simulink library "Feeder3_lib"  (Simulink 8.1)
settings: Solver=ode45  StartTime=0.0  StopTime=10.0  RelTol=1e-3
values from neighbouring files (symbols this model uses):
  Ts = 100E-6    (= 0.0001)    [BANSHEE_init.m]
undefined symbols (not defined in the file or in its folder): Left, type, V
libraries: cables_lib x14, breaker_lib x11, Load_lib x6, transformer_lib x5, powerlib x5, rtlab x3, ssn_lib x3, fault_lib x1, PQFV_lib x1, HWController_NGCHP_Genset_3p5MVA_lib x1, Motor_InductionMachine_lib x1
settings Model: Creator=re25624  LastModifiedBy=g73labuser

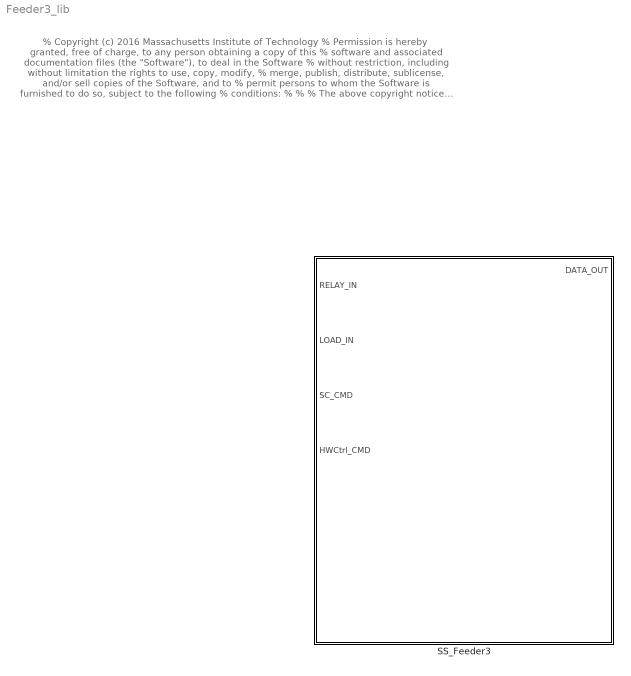
== system Feeder3_lib ==
  note: % Copyright (c) 2016 Massachusetts Institute of Technology
      | % Permission is hereby granted, free of charge, to any person obtaining a copy of this
      | % software and associated documentation files (the "Software"), to deal in the Software
      | % without restriction, including without limitation the rights to use, copy, modify,
      | % merge, publish, distribute, sublicense, and/or sell copies of the Software, and to
      | % permit persons to whom the Software is furnished to do so, subject to the following
      | % conditions:
      | %
      | %
      | % The above copyright notice and this permission notice shall be included in
      | % all copies or substantial portions of the Software.
      | %
      | % THE SOFTWARE IS PROVIDED "AS IS", WITHOUT WARRANTY OF ANY KIND, EXPRESS OR IMPLIED,
      | % INCLUDING BUT NOT LIMITED TO THE WARRANTIES OF MERCHANTABILITY, FITNESS FOR A
      | % PARTICULAR PURPOSE AND NONINFRINGEMENT. IN NO EVENT SHALL THE AUTHORS OR COPYRIGHT
      | % HOLDERS BE LIABLE FOR ANY CLAIM, DAMAGES OR OTHER LIABILITY, WHETHER IN AN ACTION
      | % OF CONTRACT, TORT OR OTHERWISE, ARISING FROM, OUT OF OR IN CONNECTION WITH THE
      | % SOFTWARE OR THE USE OR OTHER DEALINGS IN THE SOFTWARE.
      | %
      | %
      | %%
  SS_Feeder3 : Subsystem

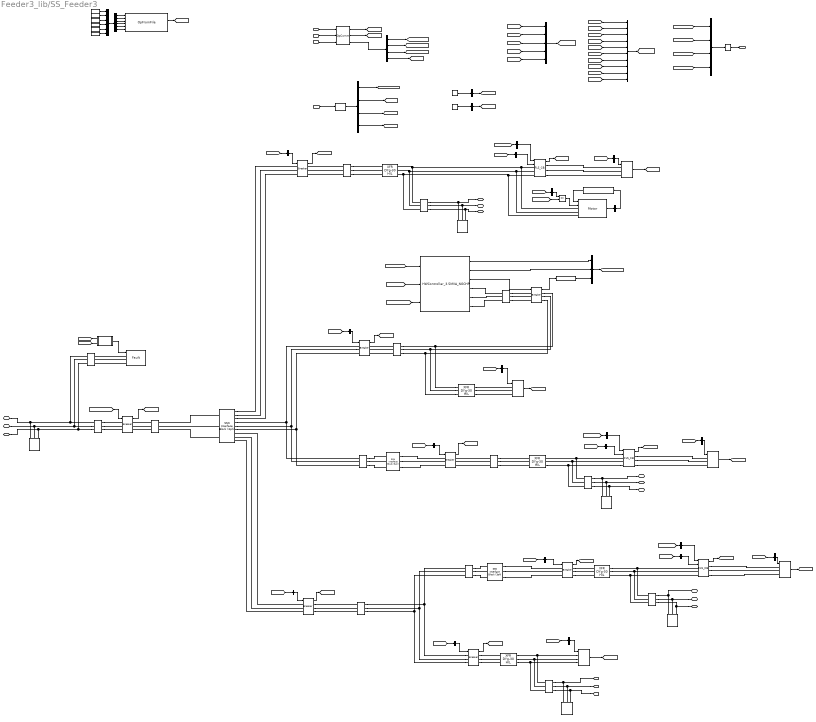
== system Feeder3_lib/SS_Feeder3 ==
  note: % Copyright (c) 2016 Massachusetts Institute of Technology
      | % Permission is hereby granted, free of charge, to any person obtaining a copy of this
      | % software and associated documentation files (the "Software"), to deal in the Software
      | % without restriction, including without limitation the rights to use, copy, modify,
      | % merge, publish, distribute, sublicense, and/or sell copies of the Software, and to
      | % permit persons to whom the Software is furnished to do so, subject to the following
      | % conditions:
      | %
      | %
      | % The above copyright notice and this permission notice shall be included in
      | % all copies or substantial portions of the Software.
      | %
      | % THE SOFTWARE IS PROVIDED "AS IS", WITHOUT WARRANTY OF ANY KIND, EXPRESS OR IMPLIED,
      | % INCLUDING BUT NOT LIMITED TO THE WARRANTIES OF MERCHANTABILITY, FITNESS FOR A
      | % PARTICULAR PURPOSE AND NONINFRINGEMENT. IN NO EVENT SHALL THE AUTHORS OR COPYRIGHT
      | % HOLDERS BE LIABLE FOR ANY CLAIM, DAMAGES OR OTHER LIABILITY, WHETHER IN AN ACTION
      | % OF CONTRACT, TORT OR OTHERWISE, ARISING FROM, OUT OF OR IN CONNECTION WITH THE
      | % SOFTWARE OR THE USE OR OTHER DEALINGS IN THE SOFTWARE.
      | %
      | %
      | %%
  note: connect to F1
  note: connect to F2
  note: connect to F2
  note: connect to F2
  note: Signal for this Cb will come from a SEL relay
  RELAY_IN : Inport
  LOAD_IN : Inport  Port=2
  SC_CMD : Inport  Port=3
  HWCtrl_CMD : Inport  Port=4
  1000 kVA : transformer_lib/XFR DYg-30 HIL  Rating=1000  Vp=13800  Vs=480  Z=5.56  XR=5.49
  1000 kVA1 : transformer_lib/XFR DYg-30 HIL  Rating=1000  Vp=13800  Vs=480  Z=5.56  XR=5.49
  200 HP chiller compressor : Load_lib/200 HP chiller compressor
  2000 kVA : transformer_lib/XFR DYg-30 HIL  Rating=2000  Vp=13800  Vs=480  Z=5.75  XR=5.7
  2000 kVA1 : transformer_lib/XFR DYg-30 HIL  Rating=2000  Vp=13800  Vs=480  Z=5.75  XR=5.7
  2500 kVA : transformer_lib/XFR DYg-30 HIL  Rating=2500  Vp=13800  Vs=480  Z=5.75  XR=6.6
  4/0AWG-Mutual : cables_lib/4//0AWG-Mutual  length=100  par_sets=1  ratio=3
  448 kvar inductor at 13.8kV  to cancel kvar produced by the stublines1 : powerlib/Elements/Three-Phase Parallel RLC Load  LConnTagsString=A|B|C  Configuration=Y (grounded)  NominalVoltage=13800  NominalFrequency=60  ActivePower=0  InductivePower=448e3  CapacitivePower=0  Measurements=None  LoadType=constant Z
  5 kvar inductor at 480V  to cancel kvar produced by the stublines : powerlib/Elements/Three-Phase Parallel RLC Load  LConnTagsString=A|B|C  Configuration=Y (grounded)  NominalVoltage=480  NominalFrequency=60  ActivePower=0  InductivePower=5e3  CapacitivePower=0  Measurements=None  LoadType=constant Z
  500kcmil-Mutual{1..2,4,7,9} (5 alike) : cables_lib/500kcmil-Mutual  length=10  par_sets=1  ratio=3
  500kcmil-Mutual3 : cables_lib/500kcmil-Mutual  length=100  par_sets=1  ratio=3
  500kcmil-Mutual5 : cables_lib/500kcmil-Mutual  length=1000  par_sets=1  ratio=3
  6 kvar inductor at 480V  to cancel kvar produced by the stublines1 : powerlib/Elements/Three-Phase Parallel RLC Load  LConnTagsString=A|B|C  Configuration=Y (grounded)  NominalVoltage=480  NominalFrequency=60  ActivePower=0  InductivePower=6e3  CapacitivePower=0  Measurements=None  LoadType=constant Z
  6 kvar inductor at 480V  to cancel kvar produced by the stublines2 : powerlib/Elements/Three-Phase Parallel RLC Load  LConnTagsString=A|B|C  Configuration=Y (grounded)  NominalVoltage=480  NominalFrequency=60  ActivePower=0  InductivePower=6e3  CapacitivePower=0  Measurements=None  LoadType=constant Z
  6 kvar inductor at 480V  to cancel kvar produced by the stublines3 : powerlib/Elements/Three-Phase Parallel RLC Load  LConnTagsString=A|B|C  Configuration=Y (grounded)  NominalVoltage=480  NominalFrequency=60  ActivePower=0  InductivePower=6e3  CapacitivePower=0  Measurements=None  LoadType=constant Z
  Bus Creator : BusCreator  Inputs=1
  Bus Creator1 : BusCreator  Inputs=1
  Bus Creator2 : BusCreator
  Bus Creator3 : BusCreator  Inputs=5
  Bus Creator5 : BusCreator  Inputs=10
  Bus Creator6 : BusCreator  Inputs=3
  Bus Selector : BusSelector  OutputSignals=motor_2
  Bus Selector1 : BusSelector  OutputSignals=F3_CB_4
  Bus Selector10 : BusSelector  OutputSignals=F3_CB_5
  Bus Selector11 : BusSelector  OutputSignals=P6
  Bus Selector12 : BusSelector  OutputSignals=F3_CB_9
  Bus Selector13 : BusSelector  OutputSignals=F3_CB_3
  Bus Selector14 : BusSelector  OutputSignals=F3_CB_8
  Bus Selector15 : BusSelector  OutputSignals=IO ctrl.16 DOUT GR3.CHP_SIM_Cmds,motor_ONOFF.F3_motor_ONOFF,fault_cmd,GridStatusCtrl.Grid_F3.Logic_trip
  Bus Selector16 : BusSelector  OutputSignals=HWCtrl.NGCHP_Gen1,HWCtrl.SEL751_LogicTrip.F3.Logic_trip,HWCtrl.SEL2440_FLS,TestSeq
  Bus Selector17 : BusSelector  OutputSignals=RPM
  Bus Selector18 : BusSelector  OutputSignals=CB309
  Bus Selector19 : BusSelector  OutputSignals=CB307
  Bus Selector2 : BusSelector  OutputSignals=C6
  Bus Selector20 : BusSelector  OutputSignals=CB308
  Bus Selector3 : BusSelector  OutputSignals=P4
  Bus Selector4 : BusSelector  OutputSignals=I6
  Bus Selector5 : BusSelector  OutputSignals=C5
  Bus Selector6 : BusSelector  OutputSignals=F3_CB_2
  Bus Selector7 : BusSelector  OutputSignals=F3_CB_7
  Bus Selector8 : BusSelector  OutputSignals=F3_CB_6
  Bus Selector9 : BusSelector  OutputSignals=F3_CB_1
  C1 : cables_lib/500kcmil-Mutual  length=10  par_sets=1  ratio=3
  C2 : cables_lib/500kcmil-Mutual  length=10  par_sets=1  ratio=3
  C301 : cables_lib/500kcmil-Mutual  length=2500  par_sets=1  ratio=3
  C302 : cables_lib/4//0AWG-Mutual  length=2000  par_sets=1  ratio=3
  C303 : cables_lib/500kcmil-Mutual  length=2000  par_sets=1  ratio=3
  C304 : cables_lib/4//0AWG-Mutual  length=1500  par_sets=2  ratio=3
  CB closed : Constant
  CB open : Constant  Value=0
  Critical_5 : Load_lib/Dynamic_Load  V=480  kVA=1000  PF=0.9  Ts=Ts
  Critical_6 : Load_lib/Dynamic_Load  V=480  kVA=800  PF=0.9  Ts=Ts
  Demux2 : Demux  Outputs=6
  F3_CB_{1..6} (6 alike) : breaker_lib/Breaker  Ts=Ts  mech_delay=cb_mech_delay
  F3_CB_7 : breaker_lib/FLS_CB  Ts=Ts  mech_delay=cb_mech_delay
  F3_CB_8 : breaker_lib/FLS_CB  Ts=Ts  mech_delay=cb_mech_delay
  F3_CB_9 : breaker_lib/FLS_CB  Ts=Ts  mech_delay=cb_mech_delay
  F3_GCB : breaker_lib/Breaker  Ts=Ts  mech_delay=cb_mech_delay
  F3_PCC : breaker_lib/Breaker  Ts=Ts  mech_delay=cb_mech_delay
  Fault_4 : fault_lib/Fault  FaultResistance=0.5  GroundResistance=1.73  SnubberResistance=1E6
  Genset_PQFV : PQFV_lib/Genset_PQFV  VRMSLL=13800  Ts=Ts
  HWController_3.5MVA_NGCHP : HWController_NGCHP_Genset_3p5MVA_lib/HWController_3.5MVA_NGCHP
  "Interpolation " : Constant
  Interruptible_6 : Load_lib/Dynamic_Load  V=480  kVA=600  PF=0.9  Ts=Ts
  Logical Operator : Logic  Operator=OR  AllPortsSameDT=off  OutDataTypeStr=boolean
  Memory : Memory
  Motor : Motor_InductionMachine_lib/Motor
  Mux : Mux  Inputs=6
  OpComm1 : rtlab/OpComm  nbport=3  groupe_acq=1  subsys_rate=0  st=0  Synchronization=on  Interpolation=on  Threshold=1.0  Missed_Data=off  Sim_Time=off  Samples=off  dynSigOut=off  from_console=0  warning_done=off  writeOpCommFile=off  Offset=off
  OpComm2 : rtlab/OpComm  nbport=1  groupe_acq=1  subsys_rate=0  st=0  Synchronization=on  Interpolation=on  Threshold=1.0  Missed_Data=off  Sim_Time=off  Samples=off  dynSigOut=off  from_console=1  warning_done=off  writeOpCommFile=off  Offset=off
  OpFromFile : rtlab/DataLogging/OpFromFile  filename_mode=Static (same filename all the time)  reload_mode=Next time model is paused (Real-Time)  init_file_id=0  filename=HeatLoad.mat  rtpath='./'  nrtpath='.\'  sample_time=Ts
  Priority_4 : Load_lib/Dynamic_Load  V=480  kVA=600  PF=0.9  Ts=Ts
  Priority_6 : Load_lib/Dynamic_Load  V=480  kVA=1000  PF=0.9  Ts=Ts
  "Repetative " : Constant
  SSN Interface Block (3ph)1 : ssn_lib/SSN Interface Block (3ph)  nb_phase=3  nb_port=2  p1_type=V-type(Left)  p2_type=V-type (Right)  p3_type=V-type(Left)  p4_type=V-type(Left)  p5_type=V-type(Left)  p6_type=V-type(Left)  p7_type=V-type(Left)  p8_type=V-type(Left)  p9_type=V-type(Left)  p10_type=V-type(Left)  p11_type=V-type(Left)  p12_type=V-type(Left)  p13_type=V-type(Left)  p14_type=V-type(Left)  p15_type=V-type(Left)  p16_type=V-type(Left)  I_port_shunt_resistance=1e9
  SSN Interface Block (3ph)2 : ssn_lib/SSN Interface Block (3ph)  nb_phase=3  nb_port=2  p1_type=V-type(Left)  p2_type=V-type (Right)  p3_type=V-type(Left)  p4_type=V-type(Left)  p5_type=V-type(Left)  p6_type=V-type(Left)  p7_type=V-type(Left)  p8_type=V-type(Left)  p9_type=V-type(Left)  p10_type=V-type(Left)  p11_type=V-type(Left)  p12_type=V-type(Left)  p13_type=V-type(Left)  p14_type=V-type(Left)  p15_type=V-type(Left)  p16_type=V-type(Left)  I_port_shunt_resistance=1e9
  SSN Interface Block (3ph)5 : ssn_lib/SSN Interface Block (3ph)  nb_phase=3  nb_port=4  p1_type=V-type(Left)  p2_type=V-type (Right)  p3_type=V-type (Right)  p4_type=V-type (Right)  p5_type=V-type(Left)  p6_type=V-type(Left)  p7_type=V-type(Left)  p8_type=V-type(Left)  p9_type=V-type(Left)  p10_type=V-type(Left)  p11_type=V-type(Left)  p12_type=V-type(Left)  p13_type=V-type(Left)  p14_type=V-type(Left)  p15_type=V-type(Left)  p16_type=V-type(Left)  I_port_shunt_resistance=1e9
  "Start_Index " : Constant
  "State " : Constant
  "Stop_Index " : Constant  Value=1800-1
  "Time_Scale_Factor " : Constant
  fault_signal : Subsystem
  A_CB_4 : PMIOPort  Port=1  Side=Right
  B_CB_4 : PMIOPort  Port=2  Side=Right
  C_CB_4 : PMIOPort  Port=3  Side=Right
  A_CB_5 : PMIOPort  Port=4  Side=Right
  B_CB_5 : PMIOPort  Port=5  Side=Right
  C_CB_5 : PMIOPort  Port=6  Side=Right
  A_CB_6 : PMIOPort  Port=7  Side=Right
  B_CB_6 : PMIOPort  Port=8  Side=Right
  C_CB_6 : PMIOPort  Port=9  Side=Right
  A_CB_7 : PMIOPort  Port=10  Side=Right
  B_CB_7 : PMIOPort  Port=11  Side=Right
  C_CB_7 : PMIOPort  Port=12  Side=Right
  PCC_A : PMIOPort  Port=13  Side=Left
  PCC_B : PMIOPort  Port=14  Side=Left
  PCC_C : PMIOPort  Port=15  Side=Left
  DATA_OUT : Outport
  wires:
  [motor_cmd] -> Logical Operator/2
  Bus Selector/1 -> Logical Operator/1  "<motor_2>"
  Logical Operator/1 -> Motor/2
  [TestSeq] -> Bus Selector/1
  fault_signal/1(o) -> Fault_4/1
  [fault_cmd] -> fault_signal/2(fault_sc)
  [TestSeq] -> fault_signal/1(fault_ts)
  Bus Selector16/4 -> [TestSeq]  "<TestSeq>"
  Bus Selector15/4 -> [feeder_cb]  "<Logic_trip>"
  Bus Selector20/1 -> F3_CB_8/1  "<CB308>"
  [SEL_2440_FLS] -> Bus Selector20/1
  Bus Selector19/1 -> F3_CB_7/1  "<CB307>"
  [SEL_2440_FLS] -> Bus Selector19/1
  Bus Selector18/1 -> F3_CB_9/1  "<CB309>"
  [SEL_2440_FLS] -> Bus Selector18/1
  Bus Selector16/3 -> [SEL_2440_FLS]  "<SEL2440_FLS>"
  Bus Selector16/2 -> [SEL751_F3_LogicTrip]  "<Logic_trip>"
  [motor_cmd] -> Bus Creator2/4  "MOTOR_ONOFF"
  200 HP chiller compressor/1 -> Motor/1
  Bus Selector17/1 -> 200 HP chiller compressor/1  "<RPM>"
  Motor/1 -> Bus Selector17/1
  Bus Selector15/1 -> [CHP_SIM_cmds]  "<CHP_SIM_Cmds>"
  [NG_CHP_DATA] -> Bus Creator2/3  "NG_CHP_DATA"
  [LOAD_DATA] -> Bus Creator2/2  "LOAD_DATA"
  [CB_DATA] -> Bus Creator2/1  "CB_DATA"
  Bus Creator2/1 -> Memory/1
  Bus Selector16/1 -> [NGCHP_Gen1]  "<NGCHP_Gen1>"
  OpComm1/3 -> Bus Selector16/1
  HWCtrl_CMD/1 -> OpComm1/3
  [heat_load] -> HWController_3.5MVA_NGCHP/1
  HWController_3.5MVA_NGCHP/3 -> F3_GCB/1
  [NGCHP_Gen1] -> HWController_3.5MVA_NGCHP/3
  Bus Creator6/1 -> [NG_CHP_DATA]
  [CHP_SIM_cmds] -> HWController_3.5MVA_NGCHP/2
  HWController_3.5MVA_NGCHP/1 -> Bus Creator6/1  "CHPData"
  HWController_3.5MVA_NGCHP/2 -> Bus Creator6/2  "Gen1_meas"
  Genset_PQFV/1 -> Bus Creator6/3  "NG_CHP_GCB"
  F3_GCB/1 -> Genset_PQFV/1
  Bus Selector15/3 -> [fault_cmd]  "<fault_cmd>"
  OpComm2/1 -> Bus Selector15/1
  Bus Selector15/2 -> [motor_cmd]  "<F3_motor_ONOFF>"
  "Stop_Index "/1 -> Mux/4
  "Interpolation "/1 -> Mux/6
  Mux/1 -> Demux2/1
  Demux2/2 -> OpFromFile/2
  Demux2/6 -> OpFromFile/6
  Demux2/3 -> OpFromFile/3
  "Repetative "/1 -> Mux/2
  Demux2/5 -> OpFromFile/5
  OpFromFile/2 -> [heat_load]  "Heat Load MBtu/hr"
  Demux2/4 -> OpFromFile/4
  Demux2/1 -> OpFromFile/1
  "State "/1 -> Mux/1
  "Time_Scale_Factor "/1 -> Mux/5
  "Start_Index "/1 -> Mux/3
  Memory/1 -> DATA_OUT/1
  SC_CMD/1 -> OpComm2/1
  [F3_CB_9] -> Bus Creator5/9  "F3_CB_9"
  [F3_CB_8] -> Bus Creator5/8  "F3_CB_8"
  [RELAY_IN] -> Bus Selector14/1
  Bus Selector14/1 -> F3_CB_8/2  "<F3_CB_8>"
  F3_CB_8/1 -> [F3_CB_8]
  [RELAY_IN] -> Bus Selector12/1
  Bus Selector12/1 -> F3_CB_9/2  "<F3_CB_9>"
  F3_CB_9/1 -> [F3_CB_9]
  [LOAD_P6] -> Bus Creator3/5  "F3_P6"
  Priority_6/1 -> [LOAD_P6]
  Bus Selector11/1 -> Priority_6/1  "<P6>"
  [LOAD_IN] -> Bus Selector11/1
  [F3_PCC] -> Bus Creator5/10  "F3_PCC"
  F3_PCC/1 -> [F3_PCC]
  F3_CB_7/1 -> [F3_CB_7]
  [SEL751_F3_LogicTrip] -> F3_PCC/1
  [RELAY_IN] -> Bus Selector13/1
  Bus Selector13/1 -> F3_CB_3/1  "<F3_CB_3>"
  [RELAY_IN] -> Bus Selector10/1
  Bus Selector10/1 -> F3_CB_5/1  "<F3_CB_5>"
  [RELAY_IN] -> Bus Selector9/1
  Bus Selector9/1 -> F3_CB_1/1  "<F3_CB_1>"
  [RELAY_IN] -> Bus Selector8/1
  Bus Selector8/1 -> F3_CB_6/1  "<F3_CB_6>"
  [RELAY_IN] -> Bus Selector7/1
  Bus Selector7/1 -> F3_CB_7/2  "<F3_CB_7>"
  [RELAY_IN] -> Bus Selector6/1
  Bus Selector6/1 -> F3_CB_2/1  "<F3_CB_2>"
  OpComm1/2 -> [RELAY_IN]
  RELAY_IN/1 -> OpComm1/2
  [RELAY_IN] -> Bus Selector1/1
  Bus Creator5/1 -> [CB_DATA]
  [F3_CB_4] -> Bus Creator5/4  "F3_CB_4"
  [F3_CB_2] -> Bus Creator5/2  "F3_CB_2"
  [F3_CB_3] -> Bus Creator5/3  "F3_CB_3"
  [F3_CB_6] -> Bus Creator5/6  "F3_CB_6"
  [F3_CB_7] -> Bus Creator5/7  "F3_CB_7"
  [F3_CB_5] -> Bus Creator5/5  "F3_CB_5"
  [F3_CB_1] -> Bus Creator5/1  "F3_CB_1"
  F3_CB_5/1 -> [F3_CB_5]
  F3_CB_1/1 -> [F3_CB_1]
  F3_CB_6/1 -> [F3_CB_6]
  F3_CB_2/1 -> [F3_CB_2]
  F3_CB_3/1 -> [F3_CB_3]
  F3_CB_4/1 -> [F3_CB_4]
  Bus Creator3/1 -> [LOAD_DATA]  "LOAD"
  [LOAD_P4] -> Bus Creator3/4  "F3_P4"
  [LOAD_I6] -> Bus Creator3/3  "F3_I6"
  [LOAD_C5] -> Bus Creator3/1  "F3_C5"
  [LOAD_C6] -> Bus Creator3/2  "F3_C6"
  Critical_5/1 -> [LOAD_C5]
  Interruptible_6/1 -> [LOAD_I6]
  Priority_4/1 -> [LOAD_P4]
  Critical_6/1 -> [LOAD_C6]
  Bus Selector5/1 -> Critical_5/1  "<C5>"
  Bus Selector4/1 -> Interruptible_6/1  "<I6>"
  Bus Selector3/1 -> Priority_4/1  "<P4>"
  Bus Selector2/1 -> Critical_6/1  "<C6>"
  [LOAD_IN] -> Bus Selector5/1
  [LOAD_IN] -> Bus Selector4/1
  [LOAD_IN] -> Bus Selector3/1
  [LOAD_IN] -> Bus Selector2/1
  OpComm1/1 -> [LOAD_IN]
  LOAD_IN/1 -> OpComm1/1
  CB open/1 -> Bus Creator1/1  "Logic_trip"
  Bus Selector1/1 -> F3_CB_4/1  "<F3_CB_4>"
  Bus Creator1/1 -> [cb_o]
  Bus Creator/1 -> [cb_c]
  CB closed/1 -> Bus Creator/1  "Logic_trip"
  connections:
  F3_CB_1/RConn3 -- C301/LConn3
  F3_CB_1/RConn2 -- C301/LConn2
  F3_CB_1/RConn1 -- C301/LConn1
  SSN Interface Block (3ph)1/RConn3 -- F3_CB_6/LConn3
  SSN Interface Block (3ph)1/RConn2 -- F3_CB_6/LConn2
  SSN Interface Block (3ph)1/RConn1 -- F3_CB_6/LConn1
  F3_CB_1/LConn3 -- SSN Interface Block (3ph)5/RConn9
  F3_CB_1/LConn1 -- SSN Interface Block (3ph)5/RConn7
  F3_CB_1/LConn2 -- SSN Interface Block (3ph)5/RConn8
  C2/RConn3 -- SSN Interface Block (3ph)2/LConn3
  C2/RConn1 -- SSN Interface Block (3ph)2/LConn1
  C2/RConn2 -- SSN Interface Block (3ph)2/LConn2
  SSN Interface Block (3ph)2/RConn1 -- F3_CB_2/LConn1
  SSN Interface Block (3ph)2/RConn2 -- F3_CB_2/LConn2
  SSN Interface Block (3ph)2/RConn3 -- F3_CB_2/LConn3
  500kcmil-Mutual5/LConn3 -- 500kcmil-Mutual7/LConn3 -- 448 kvar inductor at 13.8kV  to cancel kvar produced by the stublines1/LConn3 -- PCC_C/RConn1
  500kcmil-Mutual5/LConn2 -- 500kcmil-Mutual7/LConn2 -- 448 kvar inductor at 13.8kV  to cancel kvar produced by the stublines1/LConn2 -- PCC_B/RConn1
  448 kvar inductor at 13.8kV  to cancel kvar produced by the stublines1/LConn1 -- 500kcmil-Mutual5/LConn1 -- 500kcmil-Mutual7/LConn1 -- PCC_A/RConn1
  SSN Interface Block (3ph)5/LConn3 -- 500kcmil-Mutual3/RConn3
  SSN Interface Block (3ph)5/LConn2 -- 500kcmil-Mutual3/RConn2
  SSN Interface Block (3ph)5/LConn1 -- 500kcmil-Mutual3/RConn1
  C1/RConn1 -- SSN Interface Block (3ph)1/LConn1
  C1/RConn3 -- SSN Interface Block (3ph)1/LConn3
  C1/RConn2 -- SSN Interface Block (3ph)1/LConn2
  F3_CB_7/LConn3 -- 500kcmil-Mutual4/LConn3 -- 1000 kVA/RConn3
  500kcmil-Mutual5/RConn3 -- F3_PCC/LConn3
  500kcmil-Mutual5/RConn2 -- F3_PCC/LConn2
  500kcmil-Mutual5/RConn1 -- F3_PCC/LConn1
  500kcmil-Mutual3/LConn2 -- F3_PCC/RConn2
  500kcmil-Mutual3/LConn1 -- F3_PCC/RConn1
  500kcmil-Mutual3/LConn3 -- F3_PCC/RConn3
  B_CB_4/RConn1 -- 500kcmil-Mutual9/RConn2 -- 5 kvar inductor at 480V  to cancel kvar produced by the stublines/LConn2
  C_CB_4/RConn1 -- 500kcmil-Mutual9/RConn3 -- 5 kvar inductor at 480V  to cancel kvar produced by the stublines/LConn3
  A_CB_4/RConn1 -- 500kcmil-Mutual9/RConn1 -- 5 kvar inductor at 480V  to cancel kvar produced by the stublines/LConn1
  A_CB_7/RConn1 -- 500kcmil-Mutual4/RConn1 -- 6 kvar inductor at 480V  to cancel kvar produced by the stublines1/LConn1
  C_CB_7/RConn1 -- 500kcmil-Mutual4/RConn3 -- 6 kvar inductor at 480V  to cancel kvar produced by the stublines1/LConn3
  B_CB_7/RConn1 -- 500kcmil-Mutual4/RConn2 -- 6 kvar inductor at 480V  to cancel kvar produced by the stublines1/LConn2
  500kcmil-Mutual2/RConn1 -- A_CB_6/RConn1 -- 6 kvar inductor at 480V  to cancel kvar produced by the stublines2/LConn1
  C_CB_6/RConn1 -- 500kcmil-Mutual2/RConn3 -- 6 kvar inductor at 480V  to cancel kvar produced by the stublines2/LConn3
  B_CB_6/RConn1 -- 500kcmil-Mutual2/RConn2 -- 6 kvar inductor at 480V  to cancel kvar produced by the stublines2/LConn2
  C_CB_5/RConn1 -- 500kcmil-Mutual1/RConn3 -- 6 kvar inductor at 480V  to cancel kvar produced by the stublines3/LConn3
  6 kvar inductor at 480V  to cancel kvar produced by the stublines3/LConn1 -- 500kcmil-Mutual1/RConn1 -- A_CB_5/RConn1
  B_CB_5/RConn1 -- 500kcmil-Mutual1/RConn2 -- 6 kvar inductor at 480V  to cancel kvar produced by the stublines3/LConn2
  1000 kVA1/RConn3 -- Critical_6/LConn3
  1000 kVA1/RConn2 -- Critical_6/LConn2
  1000 kVA1/RConn1 -- Critical_6/LConn1
  HWController_3.5MVA_NGCHP/RConn1 -- 4/0AWG-Mutual/LConn1
  HWController_3.5MVA_NGCHP/RConn3 -- 4/0AWG-Mutual/LConn3
  HWController_3.5MVA_NGCHP/RConn2 -- 4/0AWG-Mutual/LConn2
  4/0AWG-Mutual/RConn1 -- F3_GCB/LConn1
  4/0AWG-Mutual/RConn2 -- F3_GCB/LConn2
  4/0AWG-Mutual/RConn3 -- F3_GCB/LConn3
  Fault_4/LConn1 -- 500kcmil-Mutual7/RConn1
  Fault_4/LConn3 -- 500kcmil-Mutual7/RConn3
  Fault_4/LConn2 -- 500kcmil-Mutual7/RConn2
  C303/RConn1 -- 2500 kVA/LConn1
  C303/RConn3 -- 2500 kVA/LConn3
  C303/RConn2 -- 2500 kVA/LConn2
  C303/LConn3 -- F3_CB_4/RConn3
  C303/LConn2 -- F3_CB_4/RConn2
  C303/LConn1 -- F3_CB_4/RConn1
  F3_CB_3/LConn2 -- C2/LConn2 -- SSN Interface Block (3ph)5/RConn5
  C2/LConn3 -- F3_CB_3/LConn3 -- SSN Interface Block (3ph)5/RConn6
  C2/LConn1 -- F3_CB_3/LConn1 -- SSN Interface Block (3ph)5/RConn4
  SSN Interface Block (3ph)5/RConn2 -- F3_CB_4/LConn2
  SSN Interface Block (3ph)5/RConn3 -- F3_CB_4/LConn3
  SSN Interface Block (3ph)5/RConn1 -- F3_CB_4/LConn1
  F3_CB_8/RConn3 -- Interruptible_6/LConn3
  F3_CB_8/RConn2 -- Interruptible_6/LConn2
  F3_CB_8/RConn1 -- Interruptible_6/LConn1
  F3_CB_9/RConn3 -- Priority_6/LConn3
  F3_CB_9/RConn2 -- Priority_6/LConn2
  F3_CB_9/RConn1 -- Priority_6/LConn1
  1000 kVA/RConn1 -- 500kcmil-Mutual4/LConn1 -- F3_CB_7/LConn1
  1000 kVA/RConn2 -- 500kcmil-Mutual4/LConn2 -- F3_CB_7/LConn2
  C304/RConn1 -- 1000 kVA/LConn1
  C304/RConn3 -- 1000 kVA/LConn3
  C304/RConn2 -- 1000 kVA/LConn2
  2500 kVA/RConn2 -- 500kcmil-Mutual9/LConn2 -- F3_CB_9/LConn2 -- Motor/LConn2
  2500 kVA/RConn3 -- 500kcmil-Mutual9/LConn3 -- Motor/LConn3 -- F3_CB_9/LConn3
  2500 kVA/RConn1 -- 500kcmil-Mutual9/LConn1 -- F3_CB_9/LConn1 -- Motor/LConn1
  Critical_5/LConn2 -- 500kcmil-Mutual1/LConn2 -- 2000 kVA/RConn2
  Critical_5/LConn3 -- 500kcmil-Mutual1/LConn3 -- 2000 kVA/RConn3
  Critical_5/LConn1 -- 500kcmil-Mutual1/LConn1 -- 2000 kVA/RConn1
  F3_CB_8/LConn2 -- 500kcmil-Mutual2/LConn2 -- 2000 kVA1/RConn2
  2000 kVA1/RConn3 -- F3_CB_8/LConn3 -- 500kcmil-Mutual2/LConn3
  F3_CB_8/LConn1 -- 500kcmil-Mutual2/LConn1 -- 2000 kVA1/RConn1
  F3_CB_7/RConn2 -- Priority_4/LConn2
  F3_CB_7/RConn3 -- Priority_4/LConn3
  F3_CB_7/RConn1 -- Priority_4/LConn1
  C304/LConn3 -- F3_CB_2/RConn3
  F3_CB_5/RConn3 -- 2000 kVA/LConn3
  F3_CB_5/RConn1 -- 2000 kVA/LConn1
  C302/LConn1 -- F3_CB_3/RConn1
  F3_CB_6/RConn1 -- 2000 kVA1/LConn1
  C304/LConn2 -- F3_CB_2/RConn2
  F3_CB_5/LConn2 -- C1/LConn2 -- C301/RConn2
  C302/LConn3 -- F3_CB_3/RConn3
  F3_CB_5/RConn2 -- 2000 kVA/LConn2
  1000 kVA1/LConn2 -- C302/RConn2 -- F3_GCB/RConn2
  F3_CB_6/RConn2 -- 2000 kVA1/LConn2
  1000 kVA1/LConn1 -- C302/RConn1 -- F3_GCB/RConn1
  C302/LConn2 -- F3_CB_3/RConn2
  1000 kVA1/LConn3 -- C302/RConn3 -- F3_GCB/RConn3
  C304/LConn1 -- F3_CB_2/RConn1
  F3_CB_5/LConn3 -- C1/LConn3 -- C301/RConn3
  F3_CB_6/RConn3 -- 2000 kVA1/LConn3
  F3_CB_5/LConn1 -- C1/LConn1 -- C301/RConn1

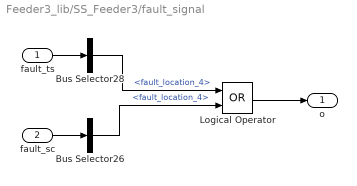
== system Feeder3_lib/SS_Feeder3/fault_signal ==
  fault_ts : Inport
  fault_sc : Inport  Port=2
  Bus Selector26 : BusSelector  OutputSignals=fault_location_4
  Bus Selector28 : BusSelector  OutputSignals=fault_location_4
  Logical Operator : Logic  Operator=OR  AllPortsSameDT=off  OutDataTypeStr=boolean
  o : Outport
  wires:
  Bus Selector28/1 -> Logical Operator/1  "<fault_location_4>"
  Logical Operator/1 -> o/1
  fault_ts/1 -> Bus Selector28/1
  Bus Selector26/1 -> Logical Operator/2  "<fault_location_4>"
  fault_sc/1 -> Bus Selector26/1
